simulink model "TD5A2017"  (R2017b)
settings: Solver=FixedStepDiscrete  StartTime=0.0  StopTime=2  FixedStep=Te  RelTol=1e-3  EnableMultiTasking=on
values from neighbouring files (symbols this model uses):
  DP = F0d.den{1}    [CorPolEx4v1.m]    (also in Exple1v1.m)
  NP = F0d.num{1}    [CorPolEx4v1.m]    (also in Exple1v1.m)
  Te = 0.72    [CorPolEx4v1.m]    (also in Exple1v1.m = 1)
undefined symbols (not defined in the file or in its folder): DPID, NPID
libraries: simulink x1
settings Model: Creator=bavisse  LastModifiedBy=lencs
settings DataIOCC: LimitDataPoints=on  SaveFormat=Array
settings OptimizationCC: LifeSpan=inf
settings DebuggingCC: SolverPrmCheckMsg=warning  SFUnexpectedBacktrackingDiag=warning  SFNoUnconditionalDefaultTransitionDiag=warning  SFExecutionAtInitializationDiag=none
settings HardwareCC: ProdBitPerPointer=32  ProdBitPerSizeT=32  ProdBitPerPtrDiffT=32  ProdLargestAtomicFloat=None  ProdIntDivRoundTo=Undefined  ProdEndianess=Unspecified  ProdWordSize=32  ProdHWDeviceType=32-bit Generic
settings ModelReferenceCC: PropagateSignalLabelsOutOfModel=off
settings CodeAppCC: StateflowObjectComments=on
settings GRTTargetCC: TargetLangStandard=C89/C90 (ANSI)  GeneratePreprocessorConditionals=Disable all
settings ConfigComp: CovMetricSettings=dw  CovHtmlReporting=on  CovSaveCumulativeToWorkspaceVar=on  CovSaveSingleToWorkspaceVar=on  CovExternalEMLEnable=off  CovSFcnEnable=off

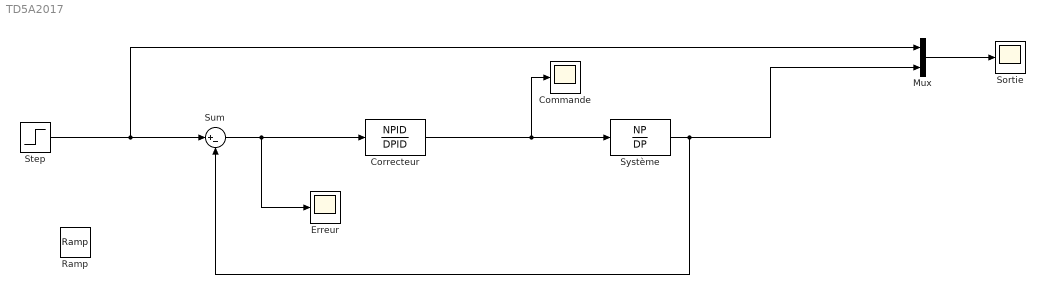
== system TD5A2017 ==
  Commande : Scope
  Correcteur : DiscreteFilter  Numerator=NPID  Denominator=DPID  SampleTime=Te  a0EqualsOne=on
  Erreur : Scope
  Mux : Mux  Inputs=2
  Ramp : simulink/Sources/Ramp  slope=1  start=0  X0=0
  Sortie : Scope
  Step : Step  SampleTime=0
  Sum : Sum  Inputs=|+-
  Système : DiscreteFilter  Numerator=NP  Denominator=DP  SampleTime=Te  a0EqualsOne=on
  wires:
  Sum/1 -> Erreur/1, Correcteur/1
  Correcteur/1 -> Commande/1, Système/1
  Système/1 -> Mux/2, Sum/2
  Mux/1 -> Sortie/1
  Step/1 -> Sum/1, Mux/1
